simulink model "punto5"  (R2022b)
settings: Solver=VariableStepAuto  StartTime=0.0  StopTime=10  RelTol=1e-3
InitFcn:
  | x0=[pi/6;0];
values from neighbouring files (symbols this model uses):
  b = 50    [Progetto_c3.m]
  e_i = 0.1    [Progetto_c3.m]
  g = 9.8    [Progetto_c3.m]
  I_e = 50    [Progetto_c3.m]
  m_i = 5    [Progetto_c3.m]
  Regolatore_totale = RR_s*RR_d    [Progetto_c3.m]
  tau_equilibrio = 1/2*g*m_i*e_i    (= 2.45)    [Progetto_c3.m]
  theta_e = pi/6    (= 0.523598775598)    [Progetto_c3.m]
settings Model: Creator=pelle  LastModifiedBy=pelle

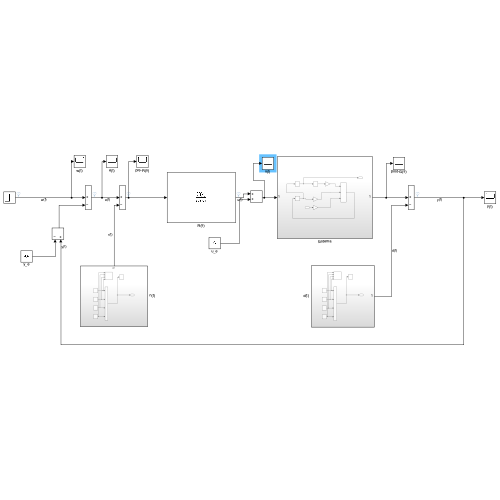
[thumbnail: Simulink's stored preview of the top-level diagram]
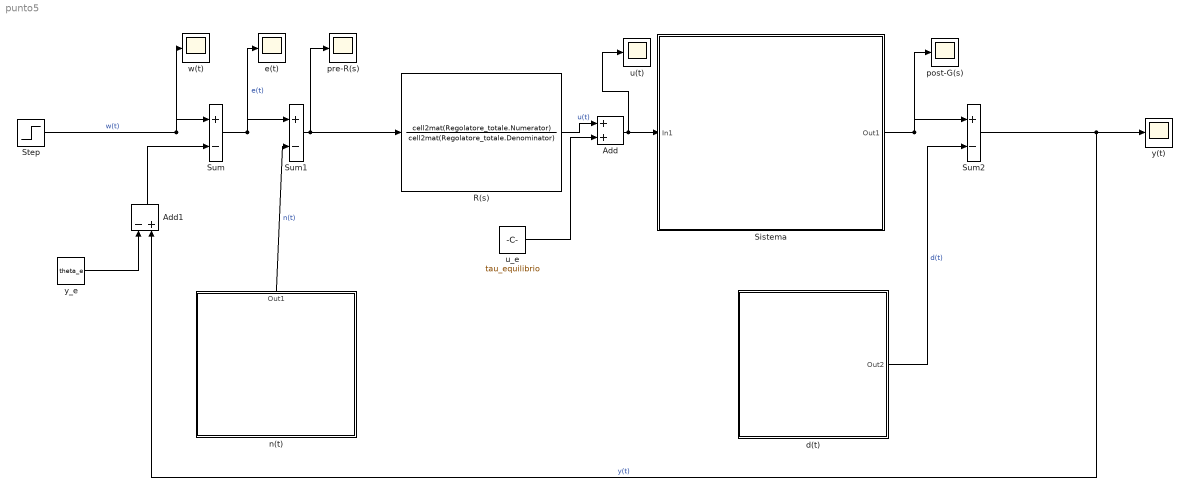
== system punto5 ==
  Add : Sum
  Add1 : Sum  Inputs=-+
  R(s) : TransferFcn  Numerator=cell2mat(Regolatore_totale.Numerator)  Denominator=cell2mat(Regolatore_totale.Denominator)
  Sistema : Subsystem
  Step : Step  Time=0  After=20  SampleTime=0
  Sum : Sum  Inputs=|+-
  Sum1 : Sum  Inputs=|+-
  Sum2 : Sum  Inputs=|+-
  d(t) : Subsystem
  e(t) : Scope
  n(t) : Subsystem
  post-G(s) : Scope
  pre-R(s) : Scope
  u(t) : Scope
  u_e : Constant  Value=tau_equilibrio
  w(t) : Scope
  y(t) : Scope
  y_e : Constant  Value=theta_e
  wires:
  Sum/1 -> e(t)/1, Sum1/1  "e(t)"
  Sum2/1 -> Add1/2, y(t)/1  "y(t)"
  n(t)/1(Out1) -> Sum1/2  "n(t)"
  Sistema/1(Out1) -> post-G(s)/1, Sum2/1
  d(t)/1(Out2) -> Sum2/2  "d(t)"
  Sum1/1 -> R(s)/1, pre-R(s)/1
  Step/1 -> w(t)/1, Sum/1  "w(t)"
  Add/1 -> u(t)/1, Sistema/1(In1)
  R(s)/1 -> Add/1  "u(t)"
  u_e/1 -> Add/2
  Add1/1 -> Sum/2
  y_e/1 -> Add1/1

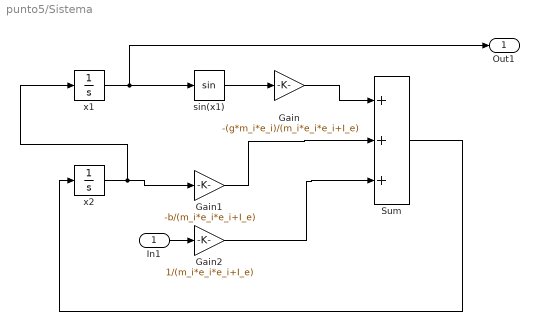
== system punto5/Sistema ==
  In1 : Inport
  Gain : Gain  Gain=-(g*m_i*e_i)/(m_i*e_i*e_i+I_e)
  Gain1 : Gain  Gain=-b/(m_i*e_i*e_i+I_e)
  Gain2 : Gain  Gain=1/(m_i*e_i*e_i+I_e)
  Sum : Sum  Inputs=+++
  sin(x1) : Trigonometry
  x1 : Integrator  InitialCondition=x0(1)
  x2 : Integrator  InitialCondition=x0(2)
  Out1 : Outport
  wires:
  In1/1 -> Gain2/1
  x1/1 -> Out1/1, sin(x1)/1
  x2/1 -> Gain1/1, x1/1
  sin(x1)/1 -> Gain/1
  Gain/1 -> Sum/1
  Gain1/1 -> Sum/2
  Gain2/1 -> Sum/3
  Sum/1 -> x2/1

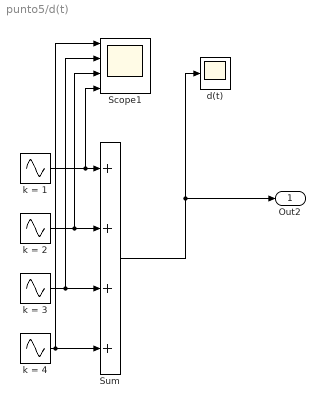
== system punto5/d(t) ==
  Scope1 : Scope  NumInputPorts=4
  Sum : Sum  Inputs=++++
  d(t) : Scope
  k = 1 : Sin  Amplitude=0.1  Frequency=1*0.025  SampleTime=0
  k = 2 : Sin  Amplitude=0.1  Frequency=2*0.025  SampleTime=0
  k = 3 : Sin  Amplitude=0.1  Frequency=3*0.025  SampleTime=0
  k = 4 : Sin  Amplitude=0.1  Frequency=4*0.025  SampleTime=0
  Out2 : Outport
  wires:
  k = 4/1 -> Scope1/1, Sum/4
  k = 1/1 -> Scope1/4, Sum/1
  k = 3/1 -> Scope1/2, Sum/3
  Sum/1 -> d(t)/1, Out2/1
  k = 2/1 -> Scope1/3, Sum/2

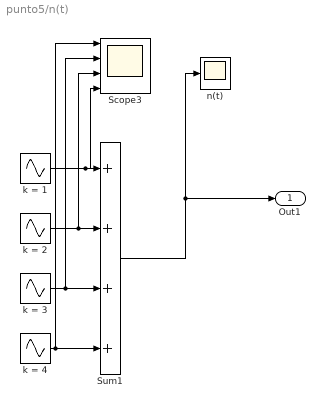
== system punto5/n(t) ==
  Scope3 : Scope  NumInputPorts=4
  Sum1 : Sum  Inputs=++++
  k = 1 : Sin  Amplitude=0.6  Frequency=1*10^3  SampleTime=0
  k = 2 : Sin  Amplitude=0.6  Frequency=2*10^3  SampleTime=0
  k = 3 : Sin  Amplitude=0.6  Frequency=3*10^3  SampleTime=0
  k = 4 : Sin  Amplitude=0.6  Frequency=4*10^3  SampleTime=0
  n(t) : Scope
  Out1 : Outport
  wires:
  k = 4/1 -> Scope3/1, Sum1/4
  k = 2/1 -> Scope3/3, Sum1/2
  Sum1/1 -> Out1/1, n(t)/1
  k = 3/1 -> Scope3/2, Sum1/3
  k = 1/1 -> Scope3/4, Sum1/1
